simulink model "system_level"  (R2023b)
settings: Solver=VariableStepAuto  StartTime=0.0  StopTime=10.0  RelTol=1e-3
libraries: eeTransforms x2
settings Model: Creator=hwma  LastModifiedBy=hwma

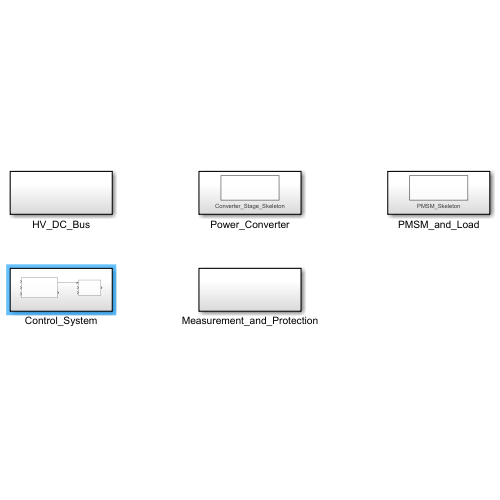
[thumbnail: Simulink's stored preview of the top-level diagram]
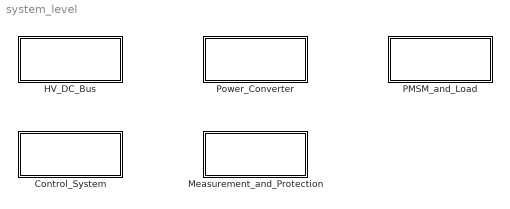
== system system_level ==
  Control_System : Subsystem
  HV_DC_Bus : Subsystem
  Measurement_and_Protection : Subsystem
  PMSM_and_Load : Subsystem
  Power_Converter : Subsystem

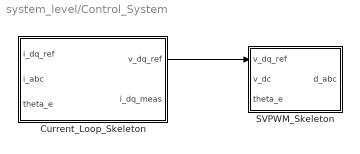
== system system_level/Control_System ==
  Current_Loop_Skeleton : Subsystem
  SVPWM_Skeleton : Subsystem
  wires:
  Current_Loop_Skeleton/1(v_dq_ref) -> SVPWM_Skeleton/1(v_dq_ref)

== system system_level/HV_DC_Bus ==

== system system_level/Measurement_and_Protection ==

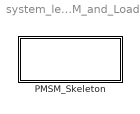
== system system_level/PMSM_and_Load ==
  PMSM_Skeleton : Subsystem

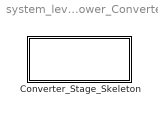
== system system_level/Power_Converter ==
  Converter_Stage_Skeleton : Subsystem

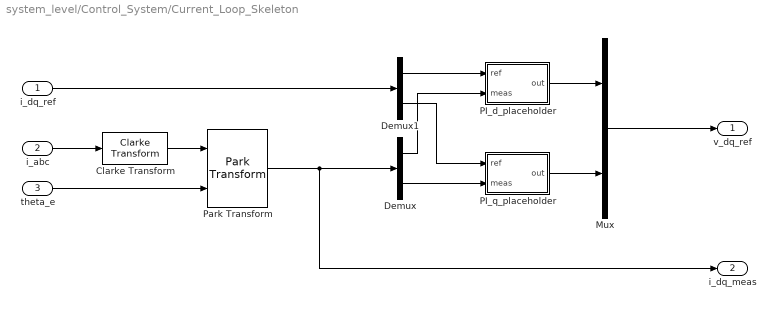
== system system_level/Control_System/Current_Loop_Skeleton ==
  i_dq_ref : Inport
  i_abc : Inport  Port=2
  theta_e : Inport  Port=3
  Clarke Transform : eeTransforms/Clarke Transform  PowerInvariant=off
      settings: LibrarySourceBlock=|
      | ee_sl_lib/Mathematical
      | Transforms/Clarke Transform
  Demux : Demux  Outputs=2
  Demux1 : Demux  Outputs=2
  Mux : Mux  Inputs=2
  PI_d_placeholder : Subsystem
  PI_q_placeholder : Subsystem
  Park Transform : eeTransforms/Park Transform  AxisAlignment=Q-axis  PowerInvariant=off
      settings: LibrarySourceBlock=|
      | ee_sl_lib/Mathematical
      | Transforms/Park Transform
  v_dq_ref : Outport
  i_dq_meas : Outport  Port=2
  wires:
  Mux/1 -> v_dq_ref/1
  PI_d_placeholder/1(out) -> Mux/1
  Clarke Transform/1 -> Park Transform/1
  theta_e/1 -> Park Transform/2
  i_abc/1 -> Clarke Transform/1
  PI_q_placeholder/1(out) -> Mux/2
  i_dq_ref/1 -> Demux1/1
  Park Transform/1 -> i_dq_meas/1, Demux/1
  Demux/2 -> PI_q_placeholder/2(meas)
  Demux1/1 -> PI_d_placeholder/1(ref)
  Demux1/2 -> PI_q_placeholder/1(ref)
  Demux/1 -> PI_d_placeholder/2(meas)

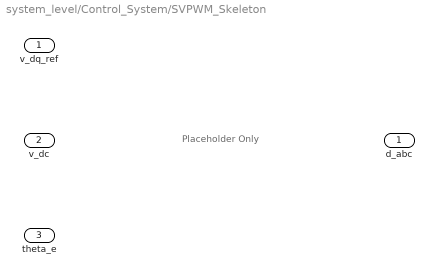
== system system_level/Control_System/SVPWM_Skeleton ==
  note: Placeholder Only
  v_dq_ref : Inport
  v_dc : Inport  Port=2
  theta_e : Inport  Port=3
  d_abc : Outport

== system system_level/PMSM_and_Load/PMSM_Skeleton ==

== system system_level/Power_Converter/Converter_Stage_Skeleton ==

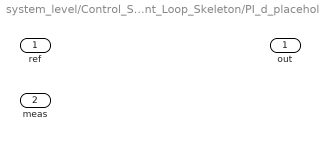
== system system_level/Control_System/Current_Loop_Skeleton/PI_d_placeholder ==
  ref : Inport
  meas : Inport  Port=2
  out : Outport

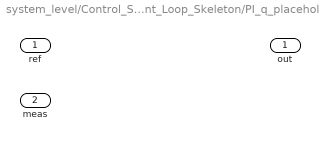
== system system_level/Control_System/Current_Loop_Skeleton/PI_q_placeholder ==
  ref : Inport
  meas : Inport  Port=2
  out : Outport
